simulink model "myqam"  (R2017a)
settings: Solver=ode45  StartTime=0.0  StopTime=10.0  RelTol=1e-3  EnableMultiTasking=on
libraries: commdigbbndam3 x2, commchan3 x1, commsink2 x1, commrflib2 x1, commrandsrc2 x1
settings Model: Creator=aa  LastModifiedBy=Administrator
settings DataIOCC: LimitDataPoints=on  SaveFormat=Array
settings OptimizationCC: LifeSpan=inf
settings DebuggingCC: SolverPrmCheckMsg=warning  SFUnexpectedBacktrackingDiag=warning  SFNoUnconditionalDefaultTransitionDiag=warning  SFExecutionAtInitializationDiag=none
settings HardwareCC: ProdBitPerPointer=32  ProdBitPerSizeT=32  ProdBitPerPtrDiffT=32  ProdLargestAtomicFloat=None  ProdIntDivRoundTo=Undefined  ProdEndianess=Unspecified  ProdWordSize=32  ProdHWDeviceType=32-bit Generic
settings ModelReferenceCC: PropagateSignalLabelsOutOfModel=off
settings GRTTargetCC: TargetLangStandard=C89/C90 (ANSI)  GeneratePreprocessorConditionals=Disable all
settings ConfigComp: CovMetricSettings=dw  CovHtmlReporting=on  CovSaveCumulativeToWorkspaceVar=on  CovSaveSingleToWorkspaceVar=on  CovExternalEMLEnable=off  CovSFcnEnable=off

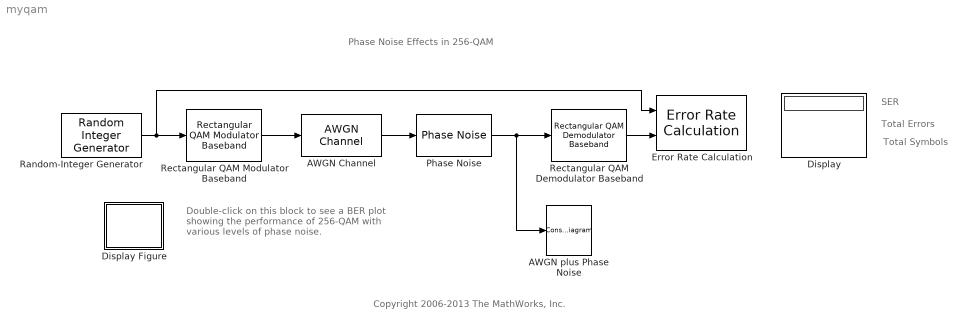
== system myqam ==
  note: Phase Noise Effects in 256-QAM
  note: Double-click on this block to see a BER plot
      | showing the performance of 256-QAM
      | with various levels of phase noise.
  note: SER
  note: Total Errors
  note: Total Symbols
  note: Copyright 2006-2013 The MathWorks, Inc.
  AWGN Channel : commchan3/AWGN Channel  InputProcessing=Columns as channels (frame based)  seed=54321  noiseMode="Signal to noise ratio  (Es/No)"  EbNodB=10  EsNodB=SNR  SNRdB=10  bitsPerSym=1  Ps=1  Tsym=.001  variance=1
  AWGN plus Phase Noise : ConstellationDiagram  Tag=ScatterPlot
  Display : Display
  Display Figure : Subsystem  mask(Display Figure){}
      settings: OpenFcn=commphasenoise_display;
      mask Display: disp('Display\nFigure');
  Error Rate Calculation : commsink2/Error Rate Calculation  N=0  st_delay=0  cp_mode=Entire frame  subframe=[]  PMode=Workspace  WsName=SER  RsMode2=off  stop=off  numErr=100  maxBits=1e6
  Phase Noise : commrflib2/Phase Noise  PhNs=PNL  Fo=1000  Fs=1024  seed=2137
      settings: SourceProductName=Communications System Toolbox  SourceProductBaseCode=CM
  Random-Integer Generator : commrandsrc2/Random Integer Generator  mul=256  seed=12345  Ts=.001  frameBased=on  sampPerFrame=500  orient=off  outDataType=uint8
  Rectangular QAM Demodulator Baseband : commdigbbndam3/Rectangular QAM Demodulator Baseband  M=256  OutType=Integer  DecType=Hard decision  VarSource=Dialog  Variance=1  Dec=Binary  Mapping=[0:15]  PowType=Average Power  MinDist=2  AvgPow=1  PeakPow=1  Ph=0  outDtype1=uint8  outDtype2=uint8  derotateFactorWordLen=16  derotateFactorDataTypeStr=Inherit: Same word length as input  derotateFactorLastDataTypeStr=Inherit: Same word length as input  denormFactorWordLen=16  denormFactorDataTypeStr=Inherit: Same word length as input  denormFactorLastDataTypeStr=Inherit: Same word length as input  prodOutWordLen=32  prodOutOverflowMode=Wrap  prodOutRoundingMode=Floor  prodOutOvFlMode=off  prodOutOvFlModeLastStrValue=off  sumWordLen=32
  Rectangular QAM Modulator Baseband : commdigbbndam3/Rectangular QAM Modulator Baseband  M=256  InType=Integer  Enc=Binary  Mapping=[0:15]  PowType=Average Power  MinDist=2  AvgPow=1  PeakPow=1  Ph=0  outDtype=single  outWordLen=16  outUDDataType=sfix(16)  outFracLenMode=Best precision  outFracLen=15  outDataTypeStr=single  outLastDataTypeStr=single
  wires:
  AWGN Channel/1 -> Phase Noise/1
  Rectangular QAM Modulator Baseband/1 -> AWGN Channel/1
  Random-Integer Generator/1 -> Rectangular QAM Modulator Baseband/1, Error Rate Calculation/1
  Phase Noise/1 -> Rectangular QAM Demodulator Baseband/1, AWGN plus Phase Noise/1
  Rectangular QAM Demodulator Baseband/1 -> Error Rate Calculation/2
  ? -> Display/1

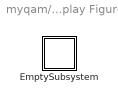
== system myqam/Display Figure ==
  EmptySubsystem : Subsystem

== system myqam/Display Figure/EmptySubsystem ==
